simulink model "Activity_99003188_2018_imp"  (R2020b)
settings: Solver=VariableStepAuto  StartTime=0.0  StopTime=10.0  RelTol=1e-3
settings Model: Creator=training  LastModifiedBy=99003188

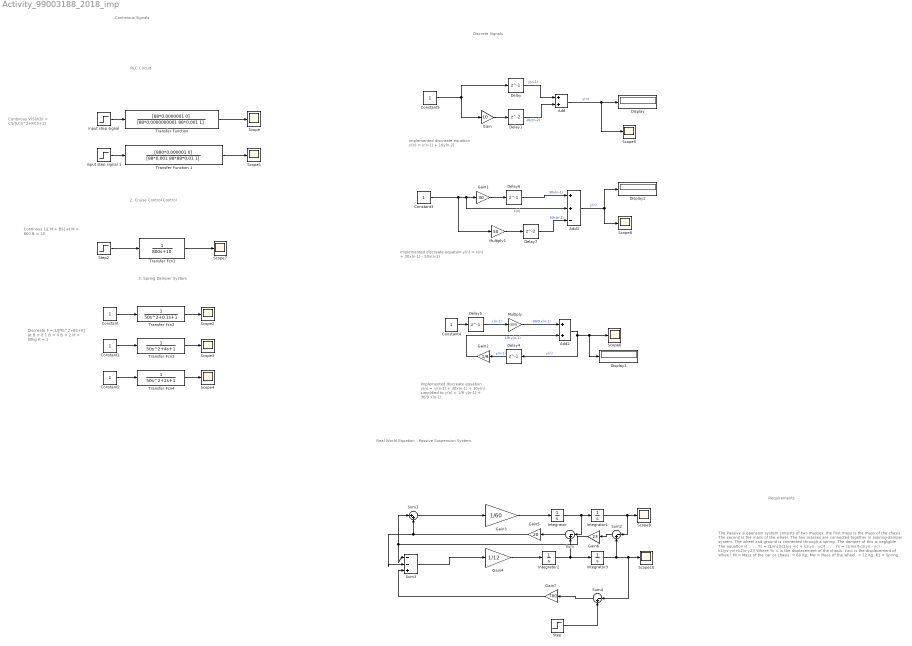
== system Activity_99003188_2018_imp ==
  note: Real World Equation : Passive Suspension System
  note: Discrete Signals
  note: 3. Spring Damper System
  note: 2. Cruise Control Control
  note: Continious Signals
  note: Continous
      | V(S)/I(S) = CS/[LCS^2+RCS+1]
  note: Discreate
      | F = 1/[MS^2+BS+K]
      | at B = 0.1
      |     B = 4
      |     B = 2
      | M = 50kg
      | K = 1
  note: Implemented discreate equation
      | y(n) = -y(n-1) + 30x(n-1) + 10y(n)
      | simplified to
      | y(n) = 1/9 y(n-1) + 30/9 x(n-1)
  note: Implemented discreate equation
      | y(n) = x(n) + 30x(n-1) - 50x(n-2)
  note: Implemented discreate equation
      | y(n) = y(n-1) + 10y(n-2)
  note: Continous
      |  	1/[ M + BS]
      | at M = 800
      |     B = 10
  note: RLC Circuit
  note: The Passive suspension system consists of two masses. the first mass is the mass of the chasis. The second is the mass of the wheel. The two masses are connected together in aspring-damper system. The wheel and ground is connected through a spring. The damper of this is negligble
      | The equation is
      | ..                        .     .
      | Yc = (1/mc)[c1(ys -yc + k1(ys - yc)]
      | ..                        .      .
      | Ys = (1/ms)[-cs(ys - yc)  - k1(ys-yc)+k2(x-y2))
      | Where
      | Yc = is the displacement of the chasis.
      | Yw= is the displacement of Whee.l
      | Mc= Mass of the car or chasis. = 60 Kg.
      | Mw = Mass of the wheel. = 12 Kg.
      | K1 = Spring coefficent between chasis and wheel = 23 N/mm
      | C1 = damper Coefficent betweem chasis and wheel = 20 Ns/mm.
      | K2 = spring between wheel and ground = 700 N/mm.
  note: Requirements
  Add : Sum
  Add2 : Sum
  Add3 : Sum  Inputs=++-
  Constant{,1..5} (6 alike) : Constant
  Delay{,4..6} (4 alike) : Delay  DelayLength=1
  Delay1 : Delay
  Delay7 : Delay
  Display : Display
  Display1 : Display
  Display2 : Display
  Gain : Gain  Gain=10
  Gain1 : Gain  Gain=30
  Gain2 : Gain  Gain=1/9
  Gain3 : Gain  Gain=1/60
  Gain4 : Gain  Gain=1/12
  Gain5 : Gain  Gain=20
  Gain6 : Gain  Gain=23
  Gain7 : Gain  Gain=700
  Integrator{,1..3} (4 alike) : Integrator
  Multiply : Gain  Gain=-30/9
  Multiply1 : Gain  Gain=50
  Scope{,1..10} (11 alike) : Scope
  Step : Step  SampleTime=0
  Step2 : Step  Time=0  SampleTime=0
  Sum : Sum  Inputs=|-+
  Sum1 : Sum  Inputs=|++
  Sum2 : Sum  Inputs=|-+
  Sum3 : Sum  Inputs=|--+
  Sum4 : Sum  Inputs=|-+
  Transfer Fcn1 : TransferFcn  Denominator=[800 10]
  Transfer Fcn2 : TransferFcn  Denominator=[50 0.1 1]
  Transfer Fcn3 : TransferFcn  Denominator=[50 4 1]
  Transfer Fcn4 : TransferFcn  Denominator=[50 2 1]
  "Transfer Function   " : TransferFcn  Numerator=[88*0.0000001 0]  Denominator=[88*0.0000000001 88*0.001 1]
  Transfer Function 1 : TransferFcn  Numerator=[880*0.000001 0]  Denominator=[88*0.001 88*88*0.01 1]
  input step signal : Step  Time=0  SampleTime=0
  "input step signal 1 " : Step  Time=0  SampleTime=0
  wires:
  "Transfer Function   "/1 -> Scope/1
  input step signal/1 -> "Transfer Function   "/1
  Constant/1 -> Transfer Fcn2/1
  Transfer Fcn2/1 -> Scope2/1
  Transfer Fcn3/1 -> Scope3/1
  Constant1/1 -> Transfer Fcn3/1
  Constant2/1 -> Transfer Fcn4/1
  Transfer Fcn4/1 -> Scope4/1
  Multiply1/1 -> Delay7/1
  Delay6/1 -> Add3/1  "30x(n-1)"
  Add3/1 -> Scope8/1, Display2/1  "y(n)"
  Constant4/1 -> Delay5/1
  Delay4/1 -> Gain2/1  "y(n-1)"
  Delay5/1 -> Multiply/1  "x(n-1)"
  Add2/1 -> Delay4/1, Display1/1, Scope6/1  "y(n)"
  Gain2/1 -> Add2/2  "1/9 y(n-1)"
  Multiply/1 -> Add2/1  "-30/9 x(n-1)"
  Constant5/1 -> Delay/1, Gain/1
  Gain/1 -> Delay1/1
  Add/1 -> Scope5/1, Display/1  "y(n)"
  Delay/1 -> Add/1  "y(n-1)"
  Delay1/1 -> Add/2  "10y(n-2)"
  Constant3/1 -> Multiply1/1, Add3/2, Gain1/1  "x(n)"
  Gain1/1 -> Delay6/1
  Delay7/1 -> Add3/3  "50x(n-2)"
  "input step signal 1 "/1 -> Transfer Function 1/1
  Transfer Function 1/1 -> Scope1/1
  Transfer Fcn1/1 -> Scope7/1
  Step2/1 -> Transfer Fcn1/1
  Gain3/1 -> Integrator/1
  Integrator/1 -> Sum/1, Integrator1/1
  Integrator1/1 -> Sum2/1, Scope9/1
  Gain4/1 -> Integrator2/1
  Integrator2/1 -> Sum/2, Integrator3/1
  Integrator3/1 -> Sum2/2, Sum4/1, Scope10/1
  Sum/1 -> Gain5/1
  Gain5/1 -> Sum3/2, Sum1/2
  Sum1/1 -> Gain3/1
  Sum2/1 -> Gain6/1
  Gain6/1 -> Sum1/1, Sum3/1
  Sum3/1 -> Gain4/1
  Sum4/1 -> Gain7/1
  Step/1 -> Sum4/2
  Gain7/1 -> Sum3/3
